simulink model "TST_APP_VD"  (R2016b)
settings: Solver=FixedStepDiscrete  StartTime=0.0  StopTime=simTime  FixedStep=sampleTime  RelTol=1e-3
values from neighbouring files (symbols this model uses):
  testCase = 1    [initTST_APP_VD_001.m]    (also in initTST_APP_VD_002.m = 2; initTST_APP_VD_003.m = 3; initTST_APP_VD_004.m = 4; initTST_APP_VD_005.m = 5)
libraries: simulink x31, UnitTest_Lib x25
settings Model: Creator=liangyunbo  LastModifiedBy=liangyunbo
settings DebuggingCC: SignalRangeChecking=error

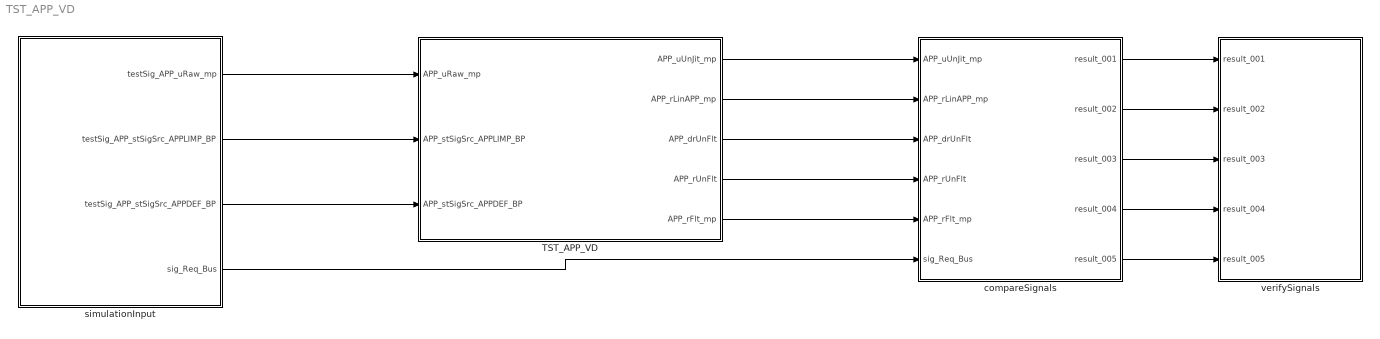
== system TST_APP_VD ==
  TST_APP_VD : Subsystem
  compareSignals : Subsystem
  simulationInput : Subsystem
  verifySignals : Subsystem
  wires:
  simulationInput/1(testSig_APP_uRaw_mp) -> TST_APP_VD/1(APP_uRaw_mp)
  simulationInput/2(testSig_APP_stSigSrc_APPLIMP_BP) -> TST_APP_VD/2(APP_stSigSrc_APPLIMP_BP)
  simulationInput/3(testSig_APP_stSigSrc_APPDEF_BP) -> TST_APP_VD/3(APP_stSigSrc_APPDEF_BP)
  TST_APP_VD/1(APP_uUnJit_mp) -> compareSignals/1(APP_uUnJit_mp)
  TST_APP_VD/2(APP_rLinAPP_mp) -> compareSignals/2(APP_rLinAPP_mp)
  TST_APP_VD/3(APP_drUnFlt) -> compareSignals/3(APP_drUnFlt)
  TST_APP_VD/4(APP_rUnFlt) -> compareSignals/4(APP_rUnFlt)
  TST_APP_VD/5(APP_rFlt_mp) -> compareSignals/5(APP_rFlt_mp)
  simulationInput/4(sig_Req_Bus) -> compareSignals/6(sig_Req_Bus)
  compareSignals/1(result_001) -> verifySignals/1(result_001)
  compareSignals/2(result_002) -> verifySignals/2(result_002)
  compareSignals/3(result_003) -> verifySignals/3(result_003)
  compareSignals/4(result_004) -> verifySignals/4(result_004)
  compareSignals/5(result_005) -> verifySignals/5(result_005)

== system TST_APP_VD/TST_APP_VD ==
  APP_uRaw_mp : Inport
  APP_stSigSrc_APPLIMP_BP : Inport  Port=2
  APP_stSigSrc_APPDEF_BP : Inport  Port=3
  APP_VD : ModelReference  ModelNameDialog=APP_VD  SimulationMode=Normal  ModelReferenceVersion=1.35  TriggerPortName=function  TriggerPortTriggerType=function-call  TriggerPortStatesWhenEnabling=held
  Function_Call : simulink/Ports & Subsystems/Function-Call Generator  sample_time=sampleTime  numberOfIterations=1
  APP_uUnJit_mp : Outport
  APP_rLinAPP_mp : Outport  Port=2
  APP_drUnFlt : Outport  Port=3
  APP_rUnFlt : Outport  Port=4
  APP_rFlt_mp : Outport  Port=5
  wires:
  Function_Call/1 -> APP_VD/Trigger
  APP_uRaw_mp/1 -> APP_VD/1
  APP_stSigSrc_APPLIMP_BP/1 -> APP_VD/2
  APP_stSigSrc_APPDEF_BP/1 -> APP_VD/3
  APP_VD/1 -> APP_uUnJit_mp/1
  APP_VD/2 -> APP_rLinAPP_mp/1
  APP_VD/3 -> APP_drUnFlt/1
  APP_VD/4 -> APP_rUnFlt/1
  APP_VD/5 -> APP_rFlt_mp/1

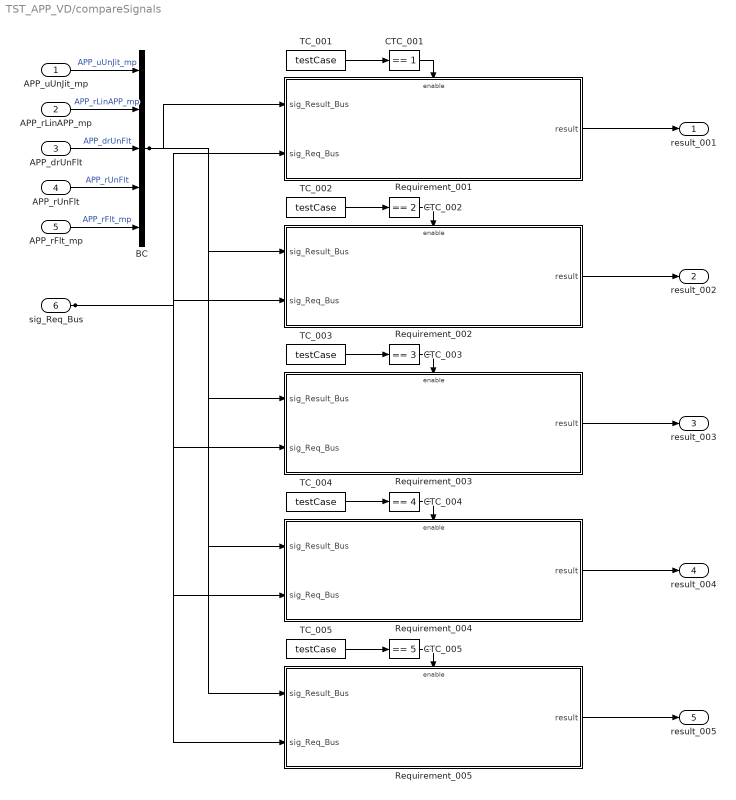
== system TST_APP_VD/compareSignals ==
  APP_uUnJit_mp : Inport
  APP_rLinAPP_mp : Inport  Port=2
  APP_drUnFlt : Inport  Port=3
  APP_rUnFlt : Inport  Port=4
  APP_rFlt_mp : Inport  Port=5
  sig_Req_Bus : Inport  Port=6
  BC : BusCreator  Inputs=5
  CTC_001 : simulink/Logic and Bit Operations/Compare To Constant  relop===  const=1  OutDataTypeStr=boolean
  CTC_002 : simulink/Logic and Bit Operations/Compare To Constant  relop===  const=2  OutDataTypeStr=boolean
  CTC_003 : simulink/Logic and Bit Operations/Compare To Constant  relop===  const=3  OutDataTypeStr=boolean
  CTC_004 : simulink/Logic and Bit Operations/Compare To Constant  relop===  const=4  OutDataTypeStr=boolean
  CTC_005 : simulink/Logic and Bit Operations/Compare To Constant  relop===  const=5  OutDataTypeStr=boolean
  Requirement_001 : Subsystem
  Requirement_002 : Subsystem
  Requirement_003 : Subsystem
  Requirement_004 : Subsystem
  Requirement_005 : Subsystem
  TC_001 : Constant  Value=testCase
  TC_002 : Constant  Value=testCase
  TC_003 : Constant  Value=testCase
  TC_004 : Constant  Value=testCase
  TC_005 : Constant  Value=testCase
  result_001 : Outport
  result_002 : Outport  Port=2
  result_003 : Outport  Port=3
  result_004 : Outport  Port=4
  result_005 : Outport  Port=5
  wires:
  APP_uUnJit_mp/1 -> BC/1  "APP_uUnJit_mp"
  APP_rLinAPP_mp/1 -> BC/2  "APP_rLinAPP_mp"
  APP_drUnFlt/1 -> BC/3  "APP_drUnFlt"
  APP_rUnFlt/1 -> BC/4  "APP_rUnFlt"
  APP_rFlt_mp/1 -> BC/5  "APP_rFlt_mp"
  TC_001/1 -> CTC_001/1
  CTC_001/1 -> Requirement_001/Enable
  sig_Req_Bus/1 -> Requirement_001/2(sig_Req_Bus), Requirement_002/2(sig_Req_Bus), Requirement_003/2(sig_Req_Bus), Requirement_004/2(sig_Req_Bus), Requirement_005/2(sig_Req_Bus)
  BC/1 -> Requirement_001/1(sig_Result_Bus), Requirement_002/1(sig_Result_Bus), Requirement_003/1(sig_Result_Bus), Requirement_004/1(sig_Result_Bus), Requirement_005/1(sig_Result_Bus)
  Requirement_001/1(result) -> result_001/1
  TC_002/1 -> CTC_002/1
  CTC_002/1 -> Requirement_002/Enable
  Requirement_002/1(result) -> result_002/1
  TC_003/1 -> CTC_003/1
  CTC_003/1 -> Requirement_003/Enable
  Requirement_003/1(result) -> result_003/1
  TC_004/1 -> CTC_004/1
  CTC_004/1 -> Requirement_004/Enable
  Requirement_004/1(result) -> result_004/1
  TC_005/1 -> CTC_005/1
  CTC_005/1 -> Requirement_005/Enable
  Requirement_005/1(result) -> result_005/1

== system TST_APP_VD/simulationInput ==
  BS : BusSelector  OutputSignals=testSig_APP_uRaw_mp,testSig_APP_stSigSrc_APPLIMP_BP,testSig_APP_stSigSrc_APPDEF_BP
  MPSw : MultiPortSwitch  Inputs=5  SaturateOnIntegerOverflow=on  InputSameDT=on
  TestCase : Constant  Value=testCase
  testSignals_R001 : Subsystem
  testSignals_R002 : Subsystem
  testSignals_R003 : Subsystem
  testSignals_R004 : Subsystem
  testSignals_R005 : Subsystem
  testSig_APP_uRaw_mp : Outport
  testSig_APP_stSigSrc_APPLIMP_BP : Outport  Port=2
  testSig_APP_stSigSrc_APPDEF_BP : Outport  Port=3
  sig_Req_Bus : Outport  Port=4
  wires:
  BS/1 -> testSig_APP_uRaw_mp/1  "<testSig_APP_uRaw_mp>"
  BS/2 -> testSig_APP_stSigSrc_APPLIMP_BP/1  "<testSig_APP_stSigSrc_APPLIMP_BP>"
  BS/3 -> testSig_APP_stSigSrc_APPDEF_BP/1  "<testSig_APP_stSigSrc_APPDEF_BP>"
  MPSw/1 -> BS/1, sig_Req_Bus/1
  TestCase/1 -> MPSw/1
  testSignals_R001/1(testSignals) -> MPSw/2
  testSignals_R002/1(testSignals) -> MPSw/3
  testSignals_R003/1(testSignals) -> MPSw/4
  testSignals_R004/1(testSignals) -> MPSw/5
  testSignals_R005/1(testSignals) -> MPSw/6

== system TST_APP_VD/verifySignals ==
  result_001 : Inport
  result_002 : Inport  Port=2
  result_003 : Inport  Port=3
  result_004 : Inport  Port=4
  result_005 : Inport  Port=5
  Assertion_001 : Assertion  Enabled=off
  Assertion_002 : Assertion  Enabled=off
  Assertion_003 : Assertion  Enabled=off
  Assertion_004 : Assertion  Enabled=off
  Assertion_005 : Assertion  Enabled=off
  wires:
  result_001/1 -> Assertion_001/1
  result_002/1 -> Assertion_002/1
  result_003/1 -> Assertion_003/1
  result_004/1 -> Assertion_004/1
  result_005/1 -> Assertion_005/1

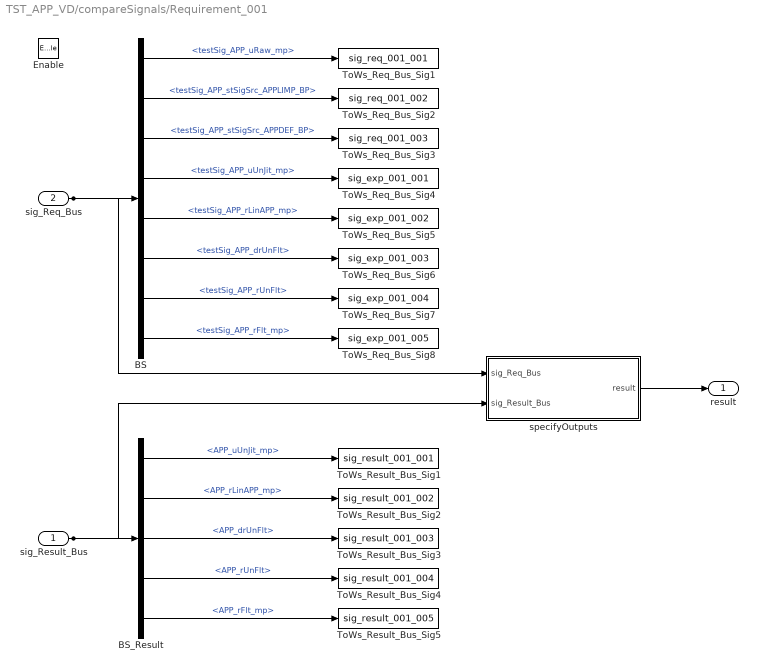
== system TST_APP_VD/compareSignals/Requirement_001 ==
  sig_Result_Bus : Inport
  sig_Req_Bus : Inport  Port=2
  Enable : EnablePort
  BS : BusSelector  OutputSignals=testSig_APP_uRaw_mp,testSig_APP_stSigSrc_APPLIMP_BP,testSig_APP_stSigSrc_APPDEF_BP,testSig_APP_uUnJit_mp,testSig_APP_rLinAPP_mp,testSig_APP_drUnFlt,testSig_APP_rUnFlt,testSig_APP_rFlt_mp
  BS_Result : BusSelector  OutputSignals=APP_uUnJit_mp,APP_rLinAPP_mp,APP_drUnFlt,APP_rUnFlt,APP_rFlt_mp
  ToWs_Req_Bus_Sig1 : ToWorkspace  VariableName=sig_req_001_001  SaveFormat=Structure With Time
  ToWs_Req_Bus_Sig2 : ToWorkspace  VariableName=sig_req_001_002  SaveFormat=Structure With Time
  ToWs_Req_Bus_Sig3 : ToWorkspace  VariableName=sig_req_001_003  SaveFormat=Structure With Time
  ToWs_Req_Bus_Sig4 : ToWorkspace  VariableName=sig_exp_001_001  SaveFormat=Structure With Time
  ToWs_Req_Bus_Sig5 : ToWorkspace  VariableName=sig_exp_001_002  SaveFormat=Structure With Time
  ToWs_Req_Bus_Sig6 : ToWorkspace  VariableName=sig_exp_001_003  SaveFormat=Structure With Time
  ToWs_Req_Bus_Sig7 : ToWorkspace  VariableName=sig_exp_001_004  SaveFormat=Structure With Time
  ToWs_Req_Bus_Sig8 : ToWorkspace  VariableName=sig_exp_001_005  SaveFormat=Structure With Time
  ToWs_Result_Bus_Sig1 : ToWorkspace  VariableName=sig_result_001_001  SaveFormat=Structure With Time
  ToWs_Result_Bus_Sig2 : ToWorkspace  VariableName=sig_result_001_002  SaveFormat=Structure With Time
  ToWs_Result_Bus_Sig3 : ToWorkspace  VariableName=sig_result_001_003  SaveFormat=Structure With Time
  ToWs_Result_Bus_Sig4 : ToWorkspace  VariableName=sig_result_001_004  SaveFormat=Structure With Time
  ToWs_Result_Bus_Sig5 : ToWorkspace  VariableName=sig_result_001_005  SaveFormat=Structure With Time
  specifyOutputs : Subsystem
  result : Outport
  wires:
  sig_Req_Bus/1 -> BS/1, specifyOutputs/1(sig_Req_Bus)
  BS/1 -> ToWs_Req_Bus_Sig1/1  "<testSig_APP_uRaw_mp>"
  BS/2 -> ToWs_Req_Bus_Sig2/1  "<testSig_APP_stSigSrc_APPLIMP_BP>"
  BS/3 -> ToWs_Req_Bus_Sig3/1  "<testSig_APP_stSigSrc_APPDEF_BP>"
  BS/4 -> ToWs_Req_Bus_Sig4/1  "<testSig_APP_uUnJit_mp>"
  BS/5 -> ToWs_Req_Bus_Sig5/1  "<testSig_APP_rLinAPP_mp>"
  BS/6 -> ToWs_Req_Bus_Sig6/1  "<testSig_APP_drUnFlt>"
  BS/7 -> ToWs_Req_Bus_Sig7/1  "<testSig_APP_rUnFlt>"
  BS/8 -> ToWs_Req_Bus_Sig8/1  "<testSig_APP_rFlt_mp>"
  sig_Result_Bus/1 -> BS_Result/1, specifyOutputs/2(sig_Result_Bus)
  BS_Result/1 -> ToWs_Result_Bus_Sig1/1  "<APP_uUnJit_mp>"
  BS_Result/2 -> ToWs_Result_Bus_Sig2/1  "<APP_rLinAPP_mp>"
  BS_Result/3 -> ToWs_Result_Bus_Sig3/1  "<APP_drUnFlt>"
  BS_Result/4 -> ToWs_Result_Bus_Sig4/1  "<APP_rUnFlt>"
  BS_Result/5 -> ToWs_Result_Bus_Sig5/1  "<APP_rFlt_mp>"
  specifyOutputs/1(result) -> result/1

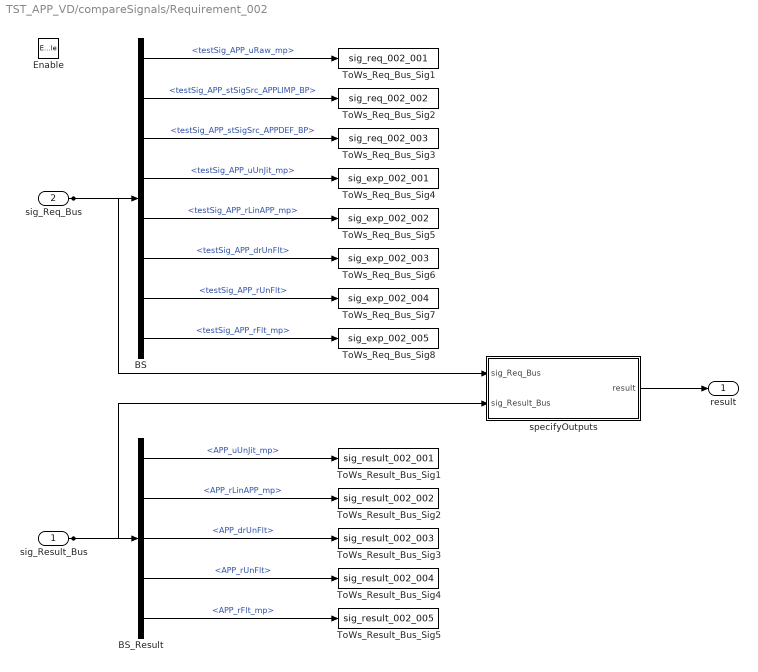
== system TST_APP_VD/compareSignals/Requirement_002 ==
  sig_Result_Bus : Inport
  sig_Req_Bus : Inport  Port=2
  Enable : EnablePort
  BS : BusSelector  OutputSignals=testSig_APP_uRaw_mp,testSig_APP_stSigSrc_APPLIMP_BP,testSig_APP_stSigSrc_APPDEF_BP,testSig_APP_uUnJit_mp,testSig_APP_rLinAPP_mp,testSig_APP_drUnFlt,testSig_APP_rUnFlt,testSig_APP_rFlt_mp
  BS_Result : BusSelector  OutputSignals=APP_uUnJit_mp,APP_rLinAPP_mp,APP_drUnFlt,APP_rUnFlt,APP_rFlt_mp
  ToWs_Req_Bus_Sig1 : ToWorkspace  VariableName=sig_req_002_001  SaveFormat=Structure With Time
  ToWs_Req_Bus_Sig2 : ToWorkspace  VariableName=sig_req_002_002  SaveFormat=Structure With Time
  ToWs_Req_Bus_Sig3 : ToWorkspace  VariableName=sig_req_002_003  SaveFormat=Structure With Time
  ToWs_Req_Bus_Sig4 : ToWorkspace  VariableName=sig_exp_002_001  SaveFormat=Structure With Time
  ToWs_Req_Bus_Sig5 : ToWorkspace  VariableName=sig_exp_002_002  SaveFormat=Structure With Time
  ToWs_Req_Bus_Sig6 : ToWorkspace  VariableName=sig_exp_002_003  SaveFormat=Structure With Time
  ToWs_Req_Bus_Sig7 : ToWorkspace  VariableName=sig_exp_002_004  SaveFormat=Structure With Time
  ToWs_Req_Bus_Sig8 : ToWorkspace  VariableName=sig_exp_002_005  SaveFormat=Structure With Time
  ToWs_Result_Bus_Sig1 : ToWorkspace  VariableName=sig_result_002_001  SaveFormat=Structure With Time
  ToWs_Result_Bus_Sig2 : ToWorkspace  VariableName=sig_result_002_002  SaveFormat=Structure With Time
  ToWs_Result_Bus_Sig3 : ToWorkspace  VariableName=sig_result_002_003  SaveFormat=Structure With Time
  ToWs_Result_Bus_Sig4 : ToWorkspace  VariableName=sig_result_002_004  SaveFormat=Structure With Time
  ToWs_Result_Bus_Sig5 : ToWorkspace  VariableName=sig_result_002_005  SaveFormat=Structure With Time
  specifyOutputs : Subsystem
  result : Outport
  wires:
  sig_Req_Bus/1 -> BS/1, specifyOutputs/1(sig_Req_Bus)
  BS/1 -> ToWs_Req_Bus_Sig1/1  "<testSig_APP_uRaw_mp>"
  BS/2 -> ToWs_Req_Bus_Sig2/1  "<testSig_APP_stSigSrc_APPLIMP_BP>"
  BS/3 -> ToWs_Req_Bus_Sig3/1  "<testSig_APP_stSigSrc_APPDEF_BP>"
  BS/4 -> ToWs_Req_Bus_Sig4/1  "<testSig_APP_uUnJit_mp>"
  BS/5 -> ToWs_Req_Bus_Sig5/1  "<testSig_APP_rLinAPP_mp>"
  BS/6 -> ToWs_Req_Bus_Sig6/1  "<testSig_APP_drUnFlt>"
  BS/7 -> ToWs_Req_Bus_Sig7/1  "<testSig_APP_rUnFlt>"
  BS/8 -> ToWs_Req_Bus_Sig8/1  "<testSig_APP_rFlt_mp>"
  sig_Result_Bus/1 -> BS_Result/1, specifyOutputs/2(sig_Result_Bus)
  BS_Result/1 -> ToWs_Result_Bus_Sig1/1  "<APP_uUnJit_mp>"
  BS_Result/2 -> ToWs_Result_Bus_Sig2/1  "<APP_rLinAPP_mp>"
  BS_Result/3 -> ToWs_Result_Bus_Sig3/1  "<APP_drUnFlt>"
  BS_Result/4 -> ToWs_Result_Bus_Sig4/1  "<APP_rUnFlt>"
  BS_Result/5 -> ToWs_Result_Bus_Sig5/1  "<APP_rFlt_mp>"
  specifyOutputs/1(result) -> result/1

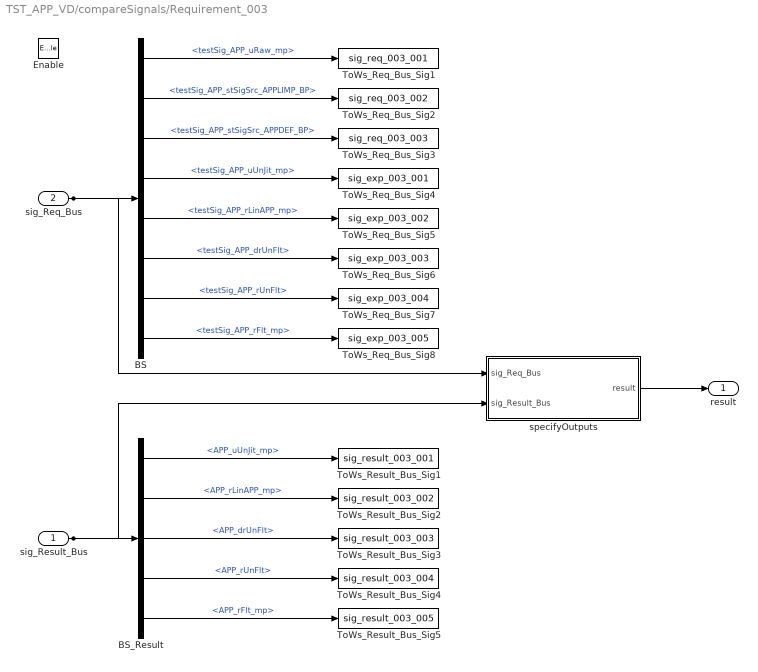
== system TST_APP_VD/compareSignals/Requirement_003 ==
  sig_Result_Bus : Inport
  sig_Req_Bus : Inport  Port=2
  Enable : EnablePort
  BS : BusSelector  OutputSignals=testSig_APP_uRaw_mp,testSig_APP_stSigSrc_APPLIMP_BP,testSig_APP_stSigSrc_APPDEF_BP,testSig_APP_uUnJit_mp,testSig_APP_rLinAPP_mp,testSig_APP_drUnFlt,testSig_APP_rUnFlt,testSig_APP_rFlt_mp
  BS_Result : BusSelector  OutputSignals=APP_uUnJit_mp,APP_rLinAPP_mp,APP_drUnFlt,APP_rUnFlt,APP_rFlt_mp
  ToWs_Req_Bus_Sig1 : ToWorkspace  VariableName=sig_req_003_001  SaveFormat=Structure With Time
  ToWs_Req_Bus_Sig2 : ToWorkspace  VariableName=sig_req_003_002  SaveFormat=Structure With Time
  ToWs_Req_Bus_Sig3 : ToWorkspace  VariableName=sig_req_003_003  SaveFormat=Structure With Time
  ToWs_Req_Bus_Sig4 : ToWorkspace  VariableName=sig_exp_003_001  SaveFormat=Structure With Time
  ToWs_Req_Bus_Sig5 : ToWorkspace  VariableName=sig_exp_003_002  SaveFormat=Structure With Time
  ToWs_Req_Bus_Sig6 : ToWorkspace  VariableName=sig_exp_003_003  SaveFormat=Structure With Time
  ToWs_Req_Bus_Sig7 : ToWorkspace  VariableName=sig_exp_003_004  SaveFormat=Structure With Time
  ToWs_Req_Bus_Sig8 : ToWorkspace  VariableName=sig_exp_003_005  SaveFormat=Structure With Time
  ToWs_Result_Bus_Sig1 : ToWorkspace  VariableName=sig_result_003_001  SaveFormat=Structure With Time
  ToWs_Result_Bus_Sig2 : ToWorkspace  VariableName=sig_result_003_002  SaveFormat=Structure With Time
  ToWs_Result_Bus_Sig3 : ToWorkspace  VariableName=sig_result_003_003  SaveFormat=Structure With Time
  ToWs_Result_Bus_Sig4 : ToWorkspace  VariableName=sig_result_003_004  SaveFormat=Structure With Time
  ToWs_Result_Bus_Sig5 : ToWorkspace  VariableName=sig_result_003_005  SaveFormat=Structure With Time
  specifyOutputs : Subsystem
  result : Outport
  wires:
  sig_Req_Bus/1 -> BS/1, specifyOutputs/1(sig_Req_Bus)
  BS/1 -> ToWs_Req_Bus_Sig1/1  "<testSig_APP_uRaw_mp>"
  BS/2 -> ToWs_Req_Bus_Sig2/1  "<testSig_APP_stSigSrc_APPLIMP_BP>"
  BS/3 -> ToWs_Req_Bus_Sig3/1  "<testSig_APP_stSigSrc_APPDEF_BP>"
  BS/4 -> ToWs_Req_Bus_Sig4/1  "<testSig_APP_uUnJit_mp>"
  BS/5 -> ToWs_Req_Bus_Sig5/1  "<testSig_APP_rLinAPP_mp>"
  BS/6 -> ToWs_Req_Bus_Sig6/1  "<testSig_APP_drUnFlt>"
  BS/7 -> ToWs_Req_Bus_Sig7/1  "<testSig_APP_rUnFlt>"
  BS/8 -> ToWs_Req_Bus_Sig8/1  "<testSig_APP_rFlt_mp>"
  sig_Result_Bus/1 -> BS_Result/1, specifyOutputs/2(sig_Result_Bus)
  BS_Result/1 -> ToWs_Result_Bus_Sig1/1  "<APP_uUnJit_mp>"
  BS_Result/2 -> ToWs_Result_Bus_Sig2/1  "<APP_rLinAPP_mp>"
  BS_Result/3 -> ToWs_Result_Bus_Sig3/1  "<APP_drUnFlt>"
  BS_Result/4 -> ToWs_Result_Bus_Sig4/1  "<APP_rUnFlt>"
  BS_Result/5 -> ToWs_Result_Bus_Sig5/1  "<APP_rFlt_mp>"
  specifyOutputs/1(result) -> result/1

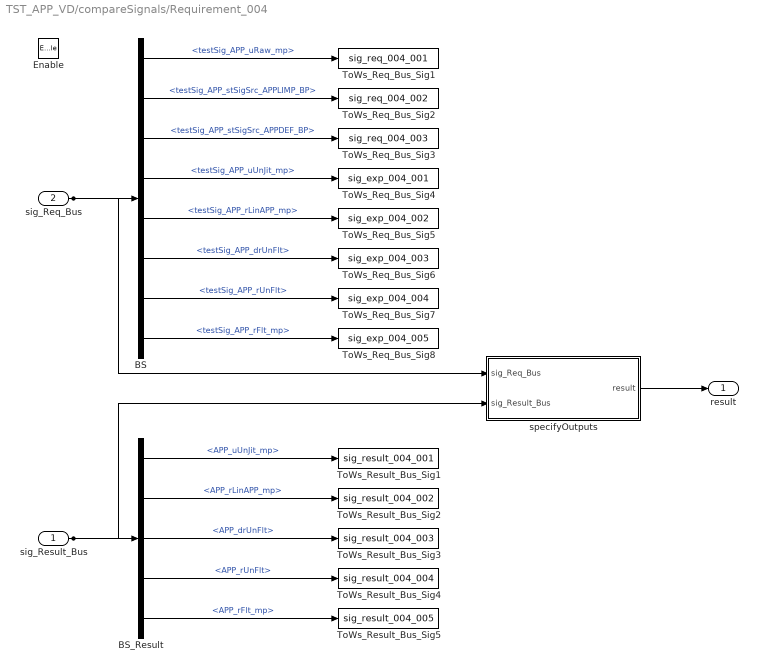
== system TST_APP_VD/compareSignals/Requirement_004 ==
  sig_Result_Bus : Inport
  sig_Req_Bus : Inport  Port=2
  Enable : EnablePort
  BS : BusSelector  OutputSignals=testSig_APP_uRaw_mp,testSig_APP_stSigSrc_APPLIMP_BP,testSig_APP_stSigSrc_APPDEF_BP,testSig_APP_uUnJit_mp,testSig_APP_rLinAPP_mp,testSig_APP_drUnFlt,testSig_APP_rUnFlt,testSig_APP_rFlt_mp
  BS_Result : BusSelector  OutputSignals=APP_uUnJit_mp,APP_rLinAPP_mp,APP_drUnFlt,APP_rUnFlt,APP_rFlt_mp
  ToWs_Req_Bus_Sig1 : ToWorkspace  VariableName=sig_req_004_001  SaveFormat=Structure With Time
  ToWs_Req_Bus_Sig2 : ToWorkspace  VariableName=sig_req_004_002  SaveFormat=Structure With Time
  ToWs_Req_Bus_Sig3 : ToWorkspace  VariableName=sig_req_004_003  SaveFormat=Structure With Time
  ToWs_Req_Bus_Sig4 : ToWorkspace  VariableName=sig_exp_004_001  SaveFormat=Structure With Time
  ToWs_Req_Bus_Sig5 : ToWorkspace  VariableName=sig_exp_004_002  SaveFormat=Structure With Time
  ToWs_Req_Bus_Sig6 : ToWorkspace  VariableName=sig_exp_004_003  SaveFormat=Structure With Time
  ToWs_Req_Bus_Sig7 : ToWorkspace  VariableName=sig_exp_004_004  SaveFormat=Structure With Time
  ToWs_Req_Bus_Sig8 : ToWorkspace  VariableName=sig_exp_004_005  SaveFormat=Structure With Time
  ToWs_Result_Bus_Sig1 : ToWorkspace  VariableName=sig_result_004_001  SaveFormat=Structure With Time
  ToWs_Result_Bus_Sig2 : ToWorkspace  VariableName=sig_result_004_002  SaveFormat=Structure With Time
  ToWs_Result_Bus_Sig3 : ToWorkspace  VariableName=sig_result_004_003  SaveFormat=Structure With Time
  ToWs_Result_Bus_Sig4 : ToWorkspace  VariableName=sig_result_004_004  SaveFormat=Structure With Time
  ToWs_Result_Bus_Sig5 : ToWorkspace  VariableName=sig_result_004_005  SaveFormat=Structure With Time
  specifyOutputs : Subsystem
  result : Outport
  wires:
  sig_Req_Bus/1 -> BS/1, specifyOutputs/1(sig_Req_Bus)
  BS/1 -> ToWs_Req_Bus_Sig1/1  "<testSig_APP_uRaw_mp>"
  BS/2 -> ToWs_Req_Bus_Sig2/1  "<testSig_APP_stSigSrc_APPLIMP_BP>"
  BS/3 -> ToWs_Req_Bus_Sig3/1  "<testSig_APP_stSigSrc_APPDEF_BP>"
  BS/4 -> ToWs_Req_Bus_Sig4/1  "<testSig_APP_uUnJit_mp>"
  BS/5 -> ToWs_Req_Bus_Sig5/1  "<testSig_APP_rLinAPP_mp>"
  BS/6 -> ToWs_Req_Bus_Sig6/1  "<testSig_APP_drUnFlt>"
  BS/7 -> ToWs_Req_Bus_Sig7/1  "<testSig_APP_rUnFlt>"
  BS/8 -> ToWs_Req_Bus_Sig8/1  "<testSig_APP_rFlt_mp>"
  sig_Result_Bus/1 -> BS_Result/1, specifyOutputs/2(sig_Result_Bus)
  BS_Result/1 -> ToWs_Result_Bus_Sig1/1  "<APP_uUnJit_mp>"
  BS_Result/2 -> ToWs_Result_Bus_Sig2/1  "<APP_rLinAPP_mp>"
  BS_Result/3 -> ToWs_Result_Bus_Sig3/1  "<APP_drUnFlt>"
  BS_Result/4 -> ToWs_Result_Bus_Sig4/1  "<APP_rUnFlt>"
  BS_Result/5 -> ToWs_Result_Bus_Sig5/1  "<APP_rFlt_mp>"
  specifyOutputs/1(result) -> result/1

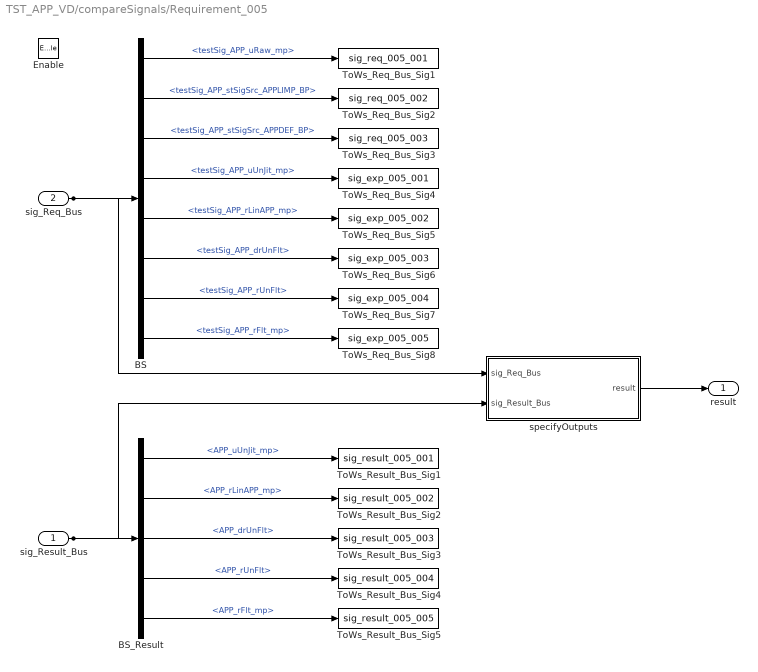
== system TST_APP_VD/compareSignals/Requirement_005 ==
  sig_Result_Bus : Inport
  sig_Req_Bus : Inport  Port=2
  Enable : EnablePort
  BS : BusSelector  OutputSignals=testSig_APP_uRaw_mp,testSig_APP_stSigSrc_APPLIMP_BP,testSig_APP_stSigSrc_APPDEF_BP,testSig_APP_uUnJit_mp,testSig_APP_rLinAPP_mp,testSig_APP_drUnFlt,testSig_APP_rUnFlt,testSig_APP_rFlt_mp
  BS_Result : BusSelector  OutputSignals=APP_uUnJit_mp,APP_rLinAPP_mp,APP_drUnFlt,APP_rUnFlt,APP_rFlt_mp
  ToWs_Req_Bus_Sig1 : ToWorkspace  VariableName=sig_req_005_001  SaveFormat=Structure With Time
  ToWs_Req_Bus_Sig2 : ToWorkspace  VariableName=sig_req_005_002  SaveFormat=Structure With Time
  ToWs_Req_Bus_Sig3 : ToWorkspace  VariableName=sig_req_005_003  SaveFormat=Structure With Time
  ToWs_Req_Bus_Sig4 : ToWorkspace  VariableName=sig_exp_005_001  SaveFormat=Structure With Time
  ToWs_Req_Bus_Sig5 : ToWorkspace  VariableName=sig_exp_005_002  SaveFormat=Structure With Time
  ToWs_Req_Bus_Sig6 : ToWorkspace  VariableName=sig_exp_005_003  SaveFormat=Structure With Time
  ToWs_Req_Bus_Sig7 : ToWorkspace  VariableName=sig_exp_005_004  SaveFormat=Structure With Time
  ToWs_Req_Bus_Sig8 : ToWorkspace  VariableName=sig_exp_005_005  SaveFormat=Structure With Time
  ToWs_Result_Bus_Sig1 : ToWorkspace  VariableName=sig_result_005_001  SaveFormat=Structure With Time
  ToWs_Result_Bus_Sig2 : ToWorkspace  VariableName=sig_result_005_002  SaveFormat=Structure With Time
  ToWs_Result_Bus_Sig3 : ToWorkspace  VariableName=sig_result_005_003  SaveFormat=Structure With Time
  ToWs_Result_Bus_Sig4 : ToWorkspace  VariableName=sig_result_005_004  SaveFormat=Structure With Time
  ToWs_Result_Bus_Sig5 : ToWorkspace  VariableName=sig_result_005_005  SaveFormat=Structure With Time
  specifyOutputs : Subsystem
  result : Outport
  wires:
  sig_Req_Bus/1 -> BS/1, specifyOutputs/1(sig_Req_Bus)
  BS/1 -> ToWs_Req_Bus_Sig1/1  "<testSig_APP_uRaw_mp>"
  BS/2 -> ToWs_Req_Bus_Sig2/1  "<testSig_APP_stSigSrc_APPLIMP_BP>"
  BS/3 -> ToWs_Req_Bus_Sig3/1  "<testSig_APP_stSigSrc_APPDEF_BP>"
  BS/4 -> ToWs_Req_Bus_Sig4/1  "<testSig_APP_uUnJit_mp>"
  BS/5 -> ToWs_Req_Bus_Sig5/1  "<testSig_APP_rLinAPP_mp>"
  BS/6 -> ToWs_Req_Bus_Sig6/1  "<testSig_APP_drUnFlt>"
  BS/7 -> ToWs_Req_Bus_Sig7/1  "<testSig_APP_rUnFlt>"
  BS/8 -> ToWs_Req_Bus_Sig8/1  "<testSig_APP_rFlt_mp>"
  sig_Result_Bus/1 -> BS_Result/1, specifyOutputs/2(sig_Result_Bus)
  BS_Result/1 -> ToWs_Result_Bus_Sig1/1  "<APP_uUnJit_mp>"
  BS_Result/2 -> ToWs_Result_Bus_Sig2/1  "<APP_rLinAPP_mp>"
  BS_Result/3 -> ToWs_Result_Bus_Sig3/1  "<APP_drUnFlt>"
  BS_Result/4 -> ToWs_Result_Bus_Sig4/1  "<APP_rUnFlt>"
  BS_Result/5 -> ToWs_Result_Bus_Sig5/1  "<APP_rFlt_mp>"
  specifyOutputs/1(result) -> result/1

== system TST_APP_VD/simulationInput/testSignals_R001 ==
  BC : BusCreator  Inputs=8
  spec_APP_drUnFlt : FromWorkspace  VariableName=testSig_APP_drUnFlt  Interpolate=off  OutputAfterFinalValue=Holding final value
  spec_APP_rFlt_mp : FromWorkspace  VariableName=testSig_APP_rFlt_mp  Interpolate=off  OutputAfterFinalValue=Holding final value
  spec_APP_rLinAPP_mp : FromWorkspace  VariableName=testSig_APP_rLinAPP_mp  Interpolate=off  OutputAfterFinalValue=Holding final value
  spec_APP_rUnFlt : FromWorkspace  VariableName=testSig_APP_rUnFlt  Interpolate=off  OutputAfterFinalValue=Holding final value
  spec_APP_stSigSrc_APPDEF_BP : FromWorkspace  VariableName=testSig_APP_stSigSrc_APPDEF_BP  Interpolate=off  OutputAfterFinalValue=Holding final value
  spec_APP_stSigSrc_APPLIMP_BP : FromWorkspace  VariableName=testSig_APP_stSigSrc_APPLIMP_BP  Interpolate=off  OutputAfterFinalValue=Holding final value
  spec_APP_uRaw_mp : FromWorkspace  VariableName=testSig_APP_uRaw_mp  Interpolate=off  OutputAfterFinalValue=Holding final value
  spec_APP_uUnJit_mp : FromWorkspace  VariableName=testSig_APP_uUnJit_mp  Interpolate=off  OutputAfterFinalValue=Holding final value
  testSignals : Outport
  wires:
  BC/1 -> testSignals/1
  spec_APP_uRaw_mp/1 -> BC/1  "testSig_APP_uRaw_mp"
  spec_APP_stSigSrc_APPLIMP_BP/1 -> BC/2  "testSig_APP_stSigSrc_APPLIMP_BP"
  spec_APP_stSigSrc_APPDEF_BP/1 -> BC/3  "testSig_APP_stSigSrc_APPDEF_BP"
  spec_APP_uUnJit_mp/1 -> BC/4  "testSig_APP_uUnJit_mp"
  spec_APP_rLinAPP_mp/1 -> BC/5  "testSig_APP_rLinAPP_mp"
  spec_APP_drUnFlt/1 -> BC/6  "testSig_APP_drUnFlt"
  spec_APP_rUnFlt/1 -> BC/7  "testSig_APP_rUnFlt"
  spec_APP_rFlt_mp/1 -> BC/8  "testSig_APP_rFlt_mp"

== system TST_APP_VD/simulationInput/testSignals_R002 ==
  BC : BusCreator  Inputs=8
  spec_APP_drUnFlt : FromWorkspace  VariableName=testSig_APP_drUnFlt  Interpolate=off  OutputAfterFinalValue=Holding final value
  spec_APP_rFlt_mp : FromWorkspace  VariableName=testSig_APP_rFlt_mp  Interpolate=off  OutputAfterFinalValue=Holding final value
  spec_APP_rLinAPP_mp : FromWorkspace  VariableName=testSig_APP_rLinAPP_mp  Interpolate=off  OutputAfterFinalValue=Holding final value
  spec_APP_rUnFlt : FromWorkspace  VariableName=testSig_APP_rUnFlt  Interpolate=off  OutputAfterFinalValue=Holding final value
  spec_APP_stSigSrc_APPDEF_BP : FromWorkspace  VariableName=testSig_APP_stSigSrc_APPDEF_BP  Interpolate=off  OutputAfterFinalValue=Holding final value
  spec_APP_stSigSrc_APPLIMP_BP : FromWorkspace  VariableName=testSig_APP_stSigSrc_APPLIMP_BP  Interpolate=off  OutputAfterFinalValue=Holding final value
  spec_APP_uRaw_mp : FromWorkspace  VariableName=testSig_APP_uRaw_mp  Interpolate=off  OutputAfterFinalValue=Holding final value
  spec_APP_uUnJit_mp : FromWorkspace  VariableName=testSig_APP_uUnJit_mp  Interpolate=off  OutputAfterFinalValue=Holding final value
  testSignals : Outport
  wires:
  BC/1 -> testSignals/1
  spec_APP_uRaw_mp/1 -> BC/1  "testSig_APP_uRaw_mp"
  spec_APP_stSigSrc_APPLIMP_BP/1 -> BC/2  "testSig_APP_stSigSrc_APPLIMP_BP"
  spec_APP_stSigSrc_APPDEF_BP/1 -> BC/3  "testSig_APP_stSigSrc_APPDEF_BP"
  spec_APP_uUnJit_mp/1 -> BC/4  "testSig_APP_uUnJit_mp"
  spec_APP_rLinAPP_mp/1 -> BC/5  "testSig_APP_rLinAPP_mp"
  spec_APP_drUnFlt/1 -> BC/6  "testSig_APP_drUnFlt"
  spec_APP_rUnFlt/1 -> BC/7  "testSig_APP_rUnFlt"
  spec_APP_rFlt_mp/1 -> BC/8  "testSig_APP_rFlt_mp"

== system TST_APP_VD/simulationInput/testSignals_R003 ==
  BC : BusCreator  Inputs=8
  spec_APP_drUnFlt : FromWorkspace  VariableName=testSig_APP_drUnFlt  Interpolate=off  OutputAfterFinalValue=Holding final value
  spec_APP_rFlt_mp : FromWorkspace  VariableName=testSig_APP_rFlt_mp  Interpolate=off  OutputAfterFinalValue=Holding final value
  spec_APP_rLinAPP_mp : FromWorkspace  VariableName=testSig_APP_rLinAPP_mp  Interpolate=off  OutputAfterFinalValue=Holding final value
  spec_APP_rUnFlt : FromWorkspace  VariableName=testSig_APP_rUnFlt  Interpolate=off  OutputAfterFinalValue=Holding final value
  spec_APP_stSigSrc_APPDEF_BP : FromWorkspace  VariableName=testSig_APP_stSigSrc_APPDEF_BP  Interpolate=off  OutputAfterFinalValue=Holding final value
  spec_APP_stSigSrc_APPLIMP_BP : FromWorkspace  VariableName=testSig_APP_stSigSrc_APPLIMP_BP  Interpolate=off  OutputAfterFinalValue=Holding final value
  spec_APP_uRaw_mp : FromWorkspace  VariableName=testSig_APP_uRaw_mp  Interpolate=off  OutputAfterFinalValue=Holding final value
  spec_APP_uUnJit_mp : FromWorkspace  VariableName=testSig_APP_uUnJit_mp  Interpolate=off  OutputAfterFinalValue=Holding final value
  testSignals : Outport
  wires:
  BC/1 -> testSignals/1
  spec_APP_uRaw_mp/1 -> BC/1  "testSig_APP_uRaw_mp"
  spec_APP_stSigSrc_APPLIMP_BP/1 -> BC/2  "testSig_APP_stSigSrc_APPLIMP_BP"
  spec_APP_stSigSrc_APPDEF_BP/1 -> BC/3  "testSig_APP_stSigSrc_APPDEF_BP"
  spec_APP_uUnJit_mp/1 -> BC/4  "testSig_APP_uUnJit_mp"
  spec_APP_rLinAPP_mp/1 -> BC/5  "testSig_APP_rLinAPP_mp"
  spec_APP_drUnFlt/1 -> BC/6  "testSig_APP_drUnFlt"
  spec_APP_rUnFlt/1 -> BC/7  "testSig_APP_rUnFlt"
  spec_APP_rFlt_mp/1 -> BC/8  "testSig_APP_rFlt_mp"

== system TST_APP_VD/simulationInput/testSignals_R004 ==
  BC : BusCreator  Inputs=8
  spec_APP_drUnFlt : FromWorkspace  VariableName=testSig_APP_drUnFlt  Interpolate=off  OutputAfterFinalValue=Holding final value
  spec_APP_rFlt_mp : FromWorkspace  VariableName=testSig_APP_rFlt_mp  Interpolate=off  OutputAfterFinalValue=Holding final value
  spec_APP_rLinAPP_mp : FromWorkspace  VariableName=testSig_APP_rLinAPP_mp  Interpolate=off  OutputAfterFinalValue=Holding final value
  spec_APP_rUnFlt : FromWorkspace  VariableName=testSig_APP_rUnFlt  Interpolate=off  OutputAfterFinalValue=Holding final value
  spec_APP_stSigSrc_APPDEF_BP : FromWorkspace  VariableName=testSig_APP_stSigSrc_APPDEF_BP  Interpolate=off  OutputAfterFinalValue=Holding final value
  spec_APP_stSigSrc_APPLIMP_BP : FromWorkspace  VariableName=testSig_APP_stSigSrc_APPLIMP_BP  Interpolate=off  OutputAfterFinalValue=Holding final value
  spec_APP_uRaw_mp : FromWorkspace  VariableName=testSig_APP_uRaw_mp  Interpolate=off  OutputAfterFinalValue=Holding final value
  spec_APP_uUnJit_mp : FromWorkspace  VariableName=testSig_APP_uUnJit_mp  Interpolate=off  OutputAfterFinalValue=Holding final value
  testSignals : Outport
  wires:
  BC/1 -> testSignals/1
  spec_APP_uRaw_mp/1 -> BC/1  "testSig_APP_uRaw_mp"
  spec_APP_stSigSrc_APPLIMP_BP/1 -> BC/2  "testSig_APP_stSigSrc_APPLIMP_BP"
  spec_APP_stSigSrc_APPDEF_BP/1 -> BC/3  "testSig_APP_stSigSrc_APPDEF_BP"
  spec_APP_uUnJit_mp/1 -> BC/4  "testSig_APP_uUnJit_mp"
  spec_APP_rLinAPP_mp/1 -> BC/5  "testSig_APP_rLinAPP_mp"
  spec_APP_drUnFlt/1 -> BC/6  "testSig_APP_drUnFlt"
  spec_APP_rUnFlt/1 -> BC/7  "testSig_APP_rUnFlt"
  spec_APP_rFlt_mp/1 -> BC/8  "testSig_APP_rFlt_mp"

== system TST_APP_VD/simulationInput/testSignals_R005 ==
  BC : BusCreator  Inputs=8
  spec_APP_drUnFlt : FromWorkspace  VariableName=testSig_APP_drUnFlt  Interpolate=off  OutputAfterFinalValue=Holding final value
  spec_APP_rFlt_mp : FromWorkspace  VariableName=testSig_APP_rFlt_mp  Interpolate=off  OutputAfterFinalValue=Holding final value
  spec_APP_rLinAPP_mp : FromWorkspace  VariableName=testSig_APP_rLinAPP_mp  Interpolate=off  OutputAfterFinalValue=Holding final value
  spec_APP_rUnFlt : FromWorkspace  VariableName=testSig_APP_rUnFlt  Interpolate=off  OutputAfterFinalValue=Holding final value
  spec_APP_stSigSrc_APPDEF_BP : FromWorkspace  VariableName=testSig_APP_stSigSrc_APPDEF_BP  Interpolate=off  OutputAfterFinalValue=Holding final value
  spec_APP_stSigSrc_APPLIMP_BP : FromWorkspace  VariableName=testSig_APP_stSigSrc_APPLIMP_BP  Interpolate=off  OutputAfterFinalValue=Holding final value
  spec_APP_uRaw_mp : FromWorkspace  VariableName=testSig_APP_uRaw_mp  Interpolate=off  OutputAfterFinalValue=Holding final value
  spec_APP_uUnJit_mp : FromWorkspace  VariableName=testSig_APP_uUnJit_mp  Interpolate=off  OutputAfterFinalValue=Holding final value
  testSignals : Outport
  wires:
  BC/1 -> testSignals/1
  spec_APP_uRaw_mp/1 -> BC/1  "testSig_APP_uRaw_mp"
  spec_APP_stSigSrc_APPLIMP_BP/1 -> BC/2  "testSig_APP_stSigSrc_APPLIMP_BP"
  spec_APP_stSigSrc_APPDEF_BP/1 -> BC/3  "testSig_APP_stSigSrc_APPDEF_BP"
  spec_APP_uUnJit_mp/1 -> BC/4  "testSig_APP_uUnJit_mp"
  spec_APP_rLinAPP_mp/1 -> BC/5  "testSig_APP_rLinAPP_mp"
  spec_APP_drUnFlt/1 -> BC/6  "testSig_APP_drUnFlt"
  spec_APP_rUnFlt/1 -> BC/7  "testSig_APP_rUnFlt"
  spec_APP_rFlt_mp/1 -> BC/8  "testSig_APP_rFlt_mp"

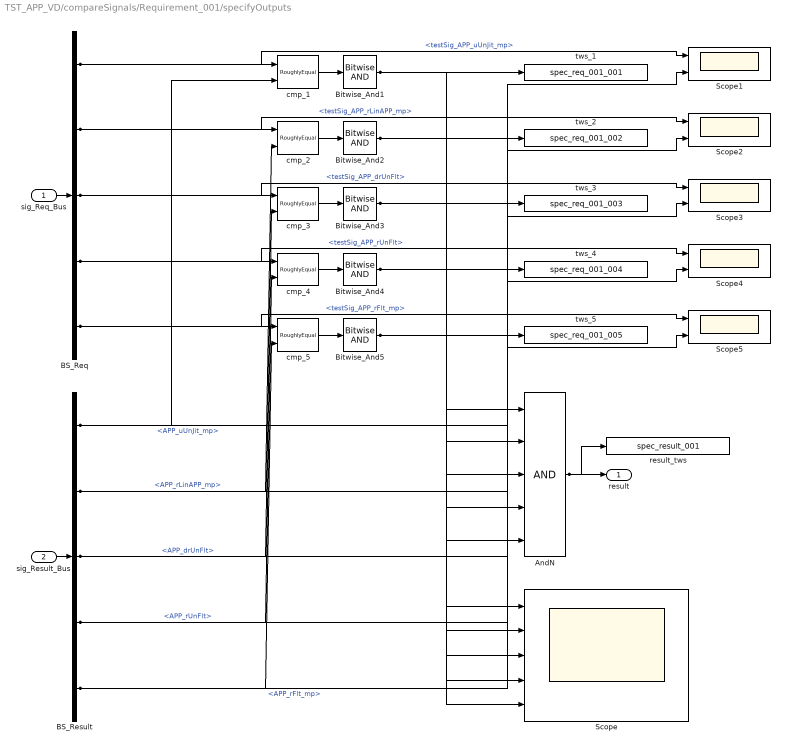
== system TST_APP_VD/compareSignals/Requirement_001/specifyOutputs ==
  sig_Req_Bus : Inport
  sig_Result_Bus : Inport  Port=2
  AndN : Logic  Inputs=5
  BS_Req : BusSelector  OutputSignals=testSig_APP_uUnJit_mp,testSig_APP_rLinAPP_mp,testSig_APP_drUnFlt,testSig_APP_rUnFlt,testSig_APP_rFlt_mp
  BS_Result : BusSelector  OutputSignals=APP_uUnJit_mp,APP_rLinAPP_mp,APP_drUnFlt,APP_rUnFlt,APP_rFlt_mp
  Bitwise_And{1..5} (5 alike) : simulink/Logic and Bit Operations/Bitwise Operator  logicop=AND  UseBitMask=off  BitMask=bin2dec('11011001')  BitMaskRealWorld=Stored Integer
  Scope : Scope  NumInputPorts=5
  Scope{1..5} (5 alike) : Scope  NumInputPorts=2
  cmp_{1..5} (5 alike) : UnitTest_Lib/RoughlyEqual  slope=0.1
  result_tws : ToWorkspace  VariableName=spec_result_001
  tws_1 : ToWorkspace  VariableName=spec_req_001_001
  tws_2 : ToWorkspace  VariableName=spec_req_001_002
  tws_3 : ToWorkspace  VariableName=spec_req_001_003
  tws_4 : ToWorkspace  VariableName=spec_req_001_004
  tws_5 : ToWorkspace  VariableName=spec_req_001_005
  result : Outport
  wires:
  sig_Req_Bus/1 -> BS_Req/1
  sig_Result_Bus/1 -> BS_Result/1
  AndN/1 -> result/1, result_tws/1
  BS_Req/1 -> cmp_1/1, Scope1/1  "<testSig_APP_uUnJit_mp>"
  BS_Result/1 -> cmp_1/2, Scope1/2  "<APP_uUnJit_mp>"
  cmp_1/1 -> Bitwise_And1/1
  Bitwise_And1/1 -> tws_1/1, AndN/1, Scope/1
  BS_Req/2 -> cmp_2/1, Scope2/1  "<testSig_APP_rLinAPP_mp>"
  BS_Result/2 -> cmp_2/2, Scope2/2  "<APP_rLinAPP_mp>"
  cmp_2/1 -> Bitwise_And2/1
  Bitwise_And2/1 -> tws_2/1, AndN/2, Scope/2
  BS_Req/3 -> cmp_3/1, Scope3/1  "<testSig_APP_drUnFlt>"
  BS_Result/3 -> cmp_3/2, Scope3/2  "<APP_drUnFlt>"
  cmp_3/1 -> Bitwise_And3/1
  Bitwise_And3/1 -> tws_3/1, AndN/3, Scope/3
  BS_Req/4 -> cmp_4/1, Scope4/1  "<testSig_APP_rUnFlt>"
  BS_Result/4 -> cmp_4/2, Scope4/2  "<APP_rUnFlt>"
  cmp_4/1 -> Bitwise_And4/1
  Bitwise_And4/1 -> tws_4/1, AndN/4, Scope/4
  BS_Req/5 -> cmp_5/1, Scope5/1  "<testSig_APP_rFlt_mp>"
  BS_Result/5 -> cmp_5/2, Scope5/2  "<APP_rFlt_mp>"
  cmp_5/1 -> Bitwise_And5/1
  Bitwise_And5/1 -> tws_5/1, AndN/5, Scope/5

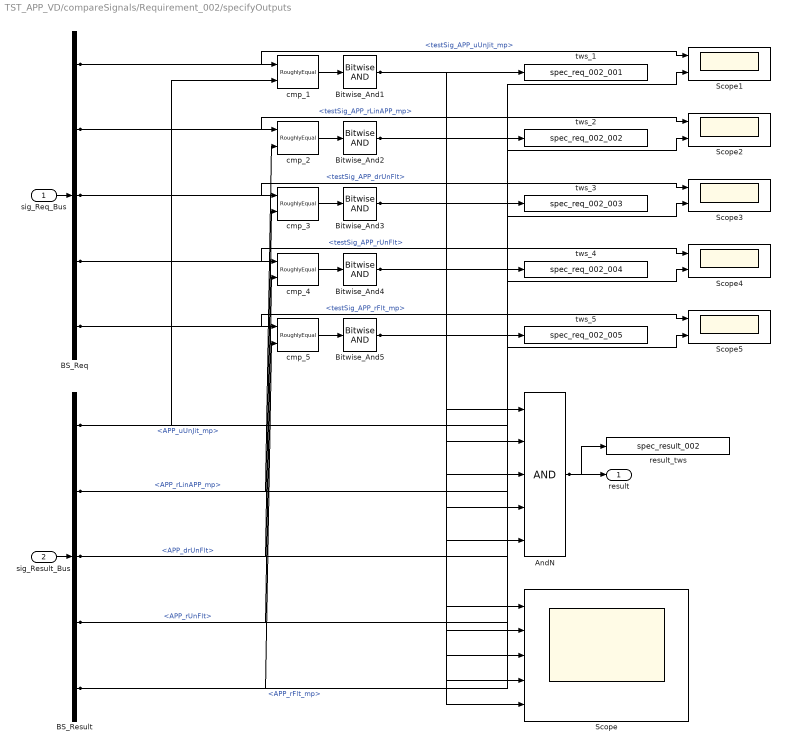
== system TST_APP_VD/compareSignals/Requirement_002/specifyOutputs ==
  sig_Req_Bus : Inport
  sig_Result_Bus : Inport  Port=2
  AndN : Logic  Inputs=5
  BS_Req : BusSelector  OutputSignals=testSig_APP_uUnJit_mp,testSig_APP_rLinAPP_mp,testSig_APP_drUnFlt,testSig_APP_rUnFlt,testSig_APP_rFlt_mp
  BS_Result : BusSelector  OutputSignals=APP_uUnJit_mp,APP_rLinAPP_mp,APP_drUnFlt,APP_rUnFlt,APP_rFlt_mp
  Bitwise_And{1..5} (5 alike) : simulink/Logic and Bit Operations/Bitwise Operator  logicop=AND  UseBitMask=off  BitMask=bin2dec('11011001')  BitMaskRealWorld=Stored Integer
  Scope : Scope  NumInputPorts=5
  Scope{1..5} (5 alike) : Scope  NumInputPorts=2
  cmp_{1..5} (5 alike) : UnitTest_Lib/RoughlyEqual  slope=0.1
  result_tws : ToWorkspace  VariableName=spec_result_002
  tws_1 : ToWorkspace  VariableName=spec_req_002_001
  tws_2 : ToWorkspace  VariableName=spec_req_002_002
  tws_3 : ToWorkspace  VariableName=spec_req_002_003
  tws_4 : ToWorkspace  VariableName=spec_req_002_004
  tws_5 : ToWorkspace  VariableName=spec_req_002_005
  result : Outport
  wires:
  sig_Req_Bus/1 -> BS_Req/1
  sig_Result_Bus/1 -> BS_Result/1
  AndN/1 -> result/1, result_tws/1
  BS_Req/1 -> cmp_1/1, Scope1/1  "<testSig_APP_uUnJit_mp>"
  BS_Result/1 -> cmp_1/2, Scope1/2  "<APP_uUnJit_mp>"
  cmp_1/1 -> Bitwise_And1/1
  Bitwise_And1/1 -> tws_1/1, AndN/1, Scope/1
  BS_Req/2 -> cmp_2/1, Scope2/1  "<testSig_APP_rLinAPP_mp>"
  BS_Result/2 -> cmp_2/2, Scope2/2  "<APP_rLinAPP_mp>"
  cmp_2/1 -> Bitwise_And2/1
  Bitwise_And2/1 -> tws_2/1, AndN/2, Scope/2
  BS_Req/3 -> cmp_3/1, Scope3/1  "<testSig_APP_drUnFlt>"
  BS_Result/3 -> cmp_3/2, Scope3/2  "<APP_drUnFlt>"
  cmp_3/1 -> Bitwise_And3/1
  Bitwise_And3/1 -> tws_3/1, AndN/3, Scope/3
  BS_Req/4 -> cmp_4/1, Scope4/1  "<testSig_APP_rUnFlt>"
  BS_Result/4 -> cmp_4/2, Scope4/2  "<APP_rUnFlt>"
  cmp_4/1 -> Bitwise_And4/1
  Bitwise_And4/1 -> tws_4/1, AndN/4, Scope/4
  BS_Req/5 -> cmp_5/1, Scope5/1  "<testSig_APP_rFlt_mp>"
  BS_Result/5 -> cmp_5/2, Scope5/2  "<APP_rFlt_mp>"
  cmp_5/1 -> Bitwise_And5/1
  Bitwise_And5/1 -> tws_5/1, AndN/5, Scope/5

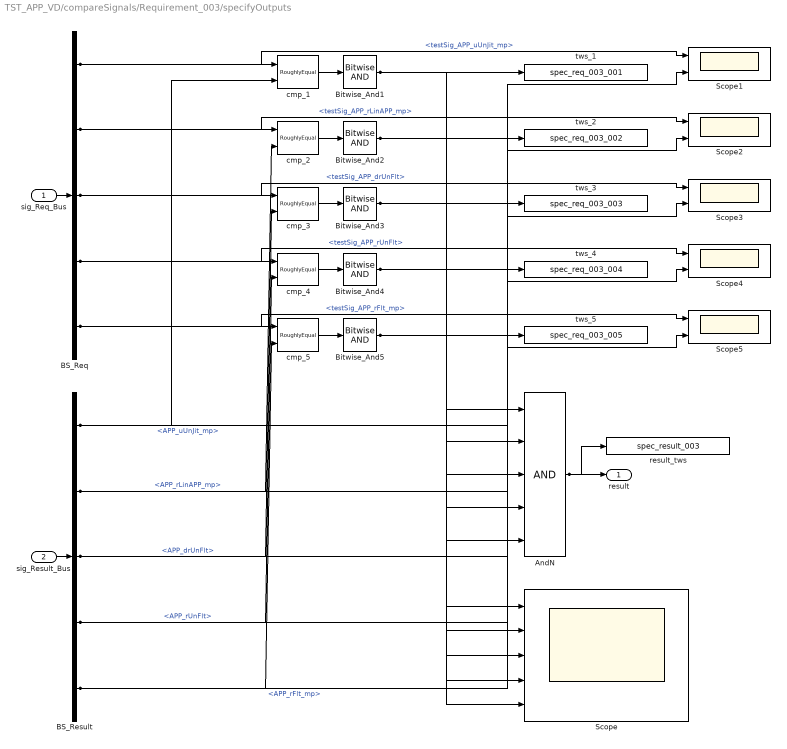
== system TST_APP_VD/compareSignals/Requirement_003/specifyOutputs ==
  sig_Req_Bus : Inport
  sig_Result_Bus : Inport  Port=2
  AndN : Logic  Inputs=5
  BS_Req : BusSelector  OutputSignals=testSig_APP_uUnJit_mp,testSig_APP_rLinAPP_mp,testSig_APP_drUnFlt,testSig_APP_rUnFlt,testSig_APP_rFlt_mp
  BS_Result : BusSelector  OutputSignals=APP_uUnJit_mp,APP_rLinAPP_mp,APP_drUnFlt,APP_rUnFlt,APP_rFlt_mp
  Bitwise_And{1..5} (5 alike) : simulink/Logic and Bit Operations/Bitwise Operator  logicop=AND  UseBitMask=off  BitMask=bin2dec('11011001')  BitMaskRealWorld=Stored Integer
  Scope : Scope  NumInputPorts=5
  Scope{1..5} (5 alike) : Scope  NumInputPorts=2
  cmp_{1..5} (5 alike) : UnitTest_Lib/RoughlyEqual  slope=0.1
  result_tws : ToWorkspace  VariableName=spec_result_003
  tws_1 : ToWorkspace  VariableName=spec_req_003_001
  tws_2 : ToWorkspace  VariableName=spec_req_003_002
  tws_3 : ToWorkspace  VariableName=spec_req_003_003
  tws_4 : ToWorkspace  VariableName=spec_req_003_004
  tws_5 : ToWorkspace  VariableName=spec_req_003_005
  result : Outport
  wires:
  sig_Req_Bus/1 -> BS_Req/1
  sig_Result_Bus/1 -> BS_Result/1
  AndN/1 -> result/1, result_tws/1
  BS_Req/1 -> cmp_1/1, Scope1/1  "<testSig_APP_uUnJit_mp>"
  BS_Result/1 -> cmp_1/2, Scope1/2  "<APP_uUnJit_mp>"
  cmp_1/1 -> Bitwise_And1/1
  Bitwise_And1/1 -> tws_1/1, AndN/1, Scope/1
  BS_Req/2 -> cmp_2/1, Scope2/1  "<testSig_APP_rLinAPP_mp>"
  BS_Result/2 -> cmp_2/2, Scope2/2  "<APP_rLinAPP_mp>"
  cmp_2/1 -> Bitwise_And2/1
  Bitwise_And2/1 -> tws_2/1, AndN/2, Scope/2
  BS_Req/3 -> cmp_3/1, Scope3/1  "<testSig_APP_drUnFlt>"
  BS_Result/3 -> cmp_3/2, Scope3/2  "<APP_drUnFlt>"
  cmp_3/1 -> Bitwise_And3/1
  Bitwise_And3/1 -> tws_3/1, AndN/3, Scope/3
  BS_Req/4 -> cmp_4/1, Scope4/1  "<testSig_APP_rUnFlt>"
  BS_Result/4 -> cmp_4/2, Scope4/2  "<APP_rUnFlt>"
  cmp_4/1 -> Bitwise_And4/1
  Bitwise_And4/1 -> tws_4/1, AndN/4, Scope/4
  BS_Req/5 -> cmp_5/1, Scope5/1  "<testSig_APP_rFlt_mp>"
  BS_Result/5 -> cmp_5/2, Scope5/2  "<APP_rFlt_mp>"
  cmp_5/1 -> Bitwise_And5/1
  Bitwise_And5/1 -> tws_5/1, AndN/5, Scope/5

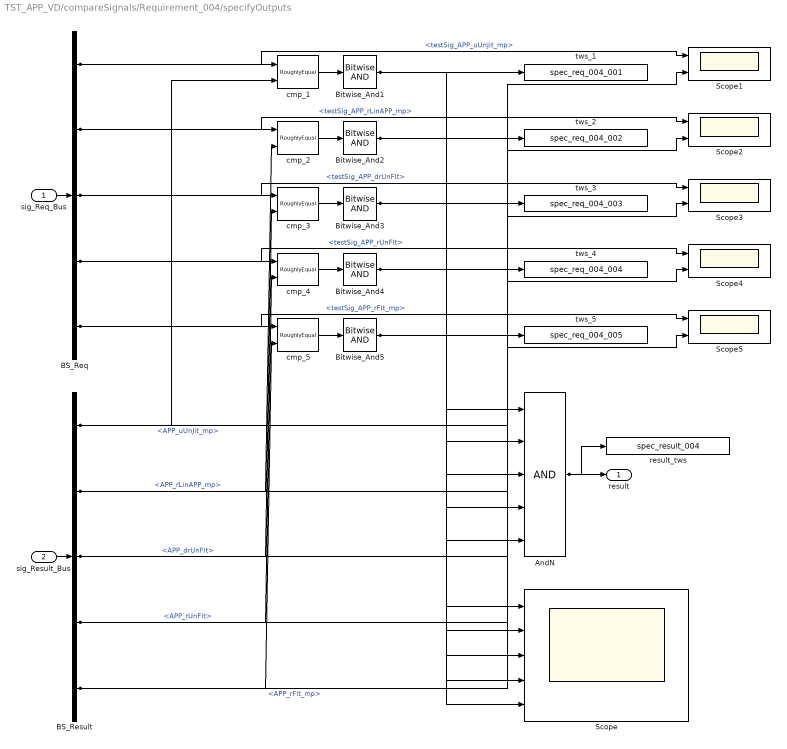
== system TST_APP_VD/compareSignals/Requirement_004/specifyOutputs ==
  sig_Req_Bus : Inport
  sig_Result_Bus : Inport  Port=2
  AndN : Logic  Inputs=5
  BS_Req : BusSelector  OutputSignals=testSig_APP_uUnJit_mp,testSig_APP_rLinAPP_mp,testSig_APP_drUnFlt,testSig_APP_rUnFlt,testSig_APP_rFlt_mp
  BS_Result : BusSelector  OutputSignals=APP_uUnJit_mp,APP_rLinAPP_mp,APP_drUnFlt,APP_rUnFlt,APP_rFlt_mp
  Bitwise_And{1..5} (5 alike) : simulink/Logic and Bit Operations/Bitwise Operator  logicop=AND  UseBitMask=off  BitMask=bin2dec('11011001')  BitMaskRealWorld=Stored Integer
  Scope : Scope  NumInputPorts=5
  Scope{1..5} (5 alike) : Scope  NumInputPorts=2
  cmp_{1..5} (5 alike) : UnitTest_Lib/RoughlyEqual  slope=0.1
  result_tws : ToWorkspace  VariableName=spec_result_004
  tws_1 : ToWorkspace  VariableName=spec_req_004_001
  tws_2 : ToWorkspace  VariableName=spec_req_004_002
  tws_3 : ToWorkspace  VariableName=spec_req_004_003
  tws_4 : ToWorkspace  VariableName=spec_req_004_004
  tws_5 : ToWorkspace  VariableName=spec_req_004_005
  result : Outport
  wires:
  sig_Req_Bus/1 -> BS_Req/1
  sig_Result_Bus/1 -> BS_Result/1
  AndN/1 -> result/1, result_tws/1
  BS_Req/1 -> cmp_1/1, Scope1/1  "<testSig_APP_uUnJit_mp>"
  BS_Result/1 -> cmp_1/2, Scope1/2  "<APP_uUnJit_mp>"
  cmp_1/1 -> Bitwise_And1/1
  Bitwise_And1/1 -> tws_1/1, AndN/1, Scope/1
  BS_Req/2 -> cmp_2/1, Scope2/1  "<testSig_APP_rLinAPP_mp>"
  BS_Result/2 -> cmp_2/2, Scope2/2  "<APP_rLinAPP_mp>"
  cmp_2/1 -> Bitwise_And2/1
  Bitwise_And2/1 -> tws_2/1, AndN/2, Scope/2
  BS_Req/3 -> cmp_3/1, Scope3/1  "<testSig_APP_drUnFlt>"
  BS_Result/3 -> cmp_3/2, Scope3/2  "<APP_drUnFlt>"
  cmp_3/1 -> Bitwise_And3/1
  Bitwise_And3/1 -> tws_3/1, AndN/3, Scope/3
  BS_Req/4 -> cmp_4/1, Scope4/1  "<testSig_APP_rUnFlt>"
  BS_Result/4 -> cmp_4/2, Scope4/2  "<APP_rUnFlt>"
  cmp_4/1 -> Bitwise_And4/1
  Bitwise_And4/1 -> tws_4/1, AndN/4, Scope/4
  BS_Req/5 -> cmp_5/1, Scope5/1  "<testSig_APP_rFlt_mp>"
  BS_Result/5 -> cmp_5/2, Scope5/2  "<APP_rFlt_mp>"
  cmp_5/1 -> Bitwise_And5/1
  Bitwise_And5/1 -> tws_5/1, AndN/5, Scope/5

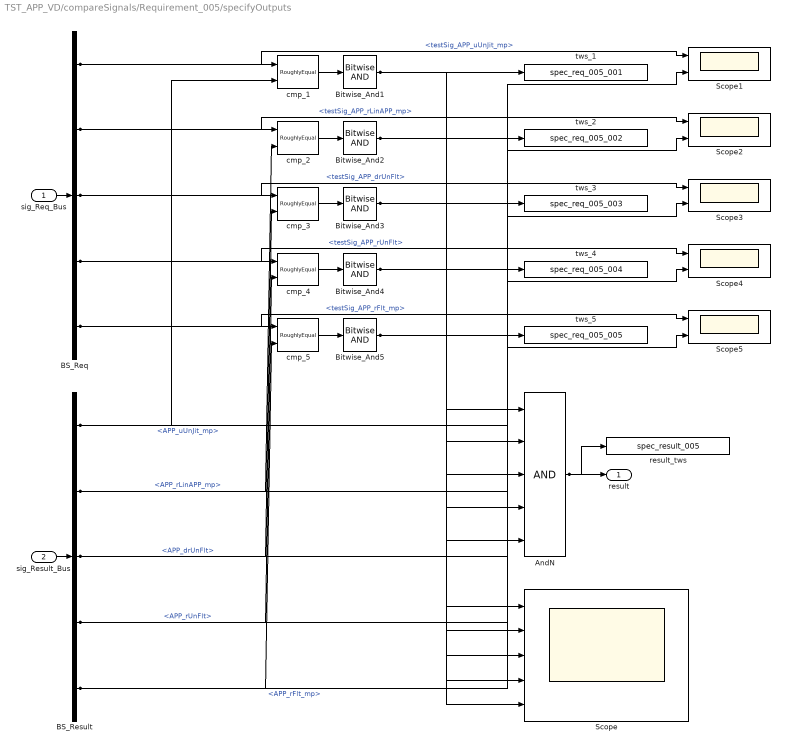
== system TST_APP_VD/compareSignals/Requirement_005/specifyOutputs ==
  sig_Req_Bus : Inport
  sig_Result_Bus : Inport  Port=2
  AndN : Logic  Inputs=5
  BS_Req : BusSelector  OutputSignals=testSig_APP_uUnJit_mp,testSig_APP_rLinAPP_mp,testSig_APP_drUnFlt,testSig_APP_rUnFlt,testSig_APP_rFlt_mp
  BS_Result : BusSelector  OutputSignals=APP_uUnJit_mp,APP_rLinAPP_mp,APP_drUnFlt,APP_rUnFlt,APP_rFlt_mp
  Bitwise_And{1..5} (5 alike) : simulink/Logic and Bit Operations/Bitwise Operator  logicop=AND  UseBitMask=off  BitMask=bin2dec('11011001')  BitMaskRealWorld=Stored Integer
  Scope : Scope  NumInputPorts=5
  Scope{1..5} (5 alike) : Scope  NumInputPorts=2
  cmp_{1..5} (5 alike) : UnitTest_Lib/RoughlyEqual  slope=0.1
  result_tws : ToWorkspace  VariableName=spec_result_005
  tws_1 : ToWorkspace  VariableName=spec_req_005_001
  tws_2 : ToWorkspace  VariableName=spec_req_005_002
  tws_3 : ToWorkspace  VariableName=spec_req_005_003
  tws_4 : ToWorkspace  VariableName=spec_req_005_004
  tws_5 : ToWorkspace  VariableName=spec_req_005_005
  result : Outport
  wires:
  sig_Req_Bus/1 -> BS_Req/1
  sig_Result_Bus/1 -> BS_Result/1
  AndN/1 -> result/1, result_tws/1
  BS_Req/1 -> cmp_1/1, Scope1/1  "<testSig_APP_uUnJit_mp>"
  BS_Result/1 -> cmp_1/2, Scope1/2  "<APP_uUnJit_mp>"
  cmp_1/1 -> Bitwise_And1/1
  Bitwise_And1/1 -> tws_1/1, AndN/1, Scope/1
  BS_Req/2 -> cmp_2/1, Scope2/1  "<testSig_APP_rLinAPP_mp>"
  BS_Result/2 -> cmp_2/2, Scope2/2  "<APP_rLinAPP_mp>"
  cmp_2/1 -> Bitwise_And2/1
  Bitwise_And2/1 -> tws_2/1, AndN/2, Scope/2
  BS_Req/3 -> cmp_3/1, Scope3/1  "<testSig_APP_drUnFlt>"
  BS_Result/3 -> cmp_3/2, Scope3/2  "<APP_drUnFlt>"
  cmp_3/1 -> Bitwise_And3/1
  Bitwise_And3/1 -> tws_3/1, AndN/3, Scope/3
  BS_Req/4 -> cmp_4/1, Scope4/1  "<testSig_APP_rUnFlt>"
  BS_Result/4 -> cmp_4/2, Scope4/2  "<APP_rUnFlt>"
  cmp_4/1 -> Bitwise_And4/1
  Bitwise_And4/1 -> tws_4/1, AndN/4, Scope/4
  BS_Req/5 -> cmp_5/1, Scope5/1  "<testSig_APP_rFlt_mp>"
  BS_Result/5 -> cmp_5/2, Scope5/2  "<APP_rFlt_mp>"
  cmp_5/1 -> Bitwise_And5/1
  Bitwise_And5/1 -> tws_5/1, AndN/5, Scope/5
